simulink model "adaptive_lms1"  (Simulink 6.6)
settings: Solver=VariableStepDiscrete  StartTime=0.0  StopTime=15  RelTol=1e-3
StartFcn:
  | tic
StopFcn:
  | toc
libraries: dspbuff3 x2, simulink x2, dspwin32 x2, dspsigops x1, dspadpt3 x1
settings Model: Creator=lcrockett  LastModifiedBy=lcrockett
settings OptimizationCC: InlineParams=on  InlineInvariantSignals=on
settings DebuggingCC: SignalResolutionControl=TryResolveAllWithWarning  MultiTaskDSMMsg=warning  MultiTaskCondExecSysMsg=none  StrictBusMsg=None
settings HardwareCC: TargetHWDeviceType=32-bit Generic  ProdEqTarget=off
settings RTWCC: IncludeERTFirstTime=on

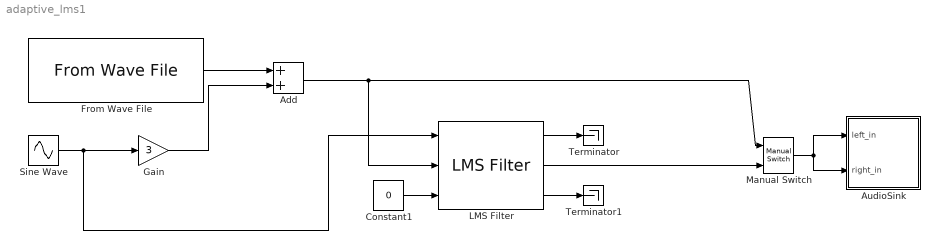
== system adaptive_lms1 ==
  Add : Sum  OutScaling=2^-10
  AudioSink : Subsystem
  Constant1 : Constant  Value=0
  From Wave File : dspwin32/From Wave File  FileName=Yabu_sample_48_mono  SamplesPerFrame=1  MinBufSize=1  dType=double  bLoop=off  timesToPlay=1  restartMode=immediately after last sample  firstSampleOutput=off  lastSampleOutput=off
  Gain : Gain  Gain=3
  LMS Filter : dspadpt3/LMS Filter  DialogController=dspDDGCreate  DialogControllerArgs=DataTag0  Algo=LMS  L=4  stepflag=Dialog  mu=0.001  leakage=1.0  ic=0  Adapt=off  resetflag=Non-zero sample  weights=on  secondCoeffMode=User-defined  secondCoeffWordLength=2  secondCoeffFracLength=15  accum2Mode=User-defined  accum2FracLength=20  prodOutput2Mode=User-defined  prodOutput2FracLength=20  prodOutput3Mode=User-defined  prodOutput3FracLength=20  prodOutput4Mode=User-defined  prodOutput4FracLength=20  quotientMode=User-defined  quotientFracLength=20  roundingMode=Floor  overflowMode=off  addnparflag=off
  Manual Switch : simulink/Signal Routing/Manual Switch  SystemSampleTime=-1  sw=0  action=0  varsize=off
  Sine Wave : Sin  Amplitude=0.5  Frequency=2*pi*1200  SampleTime=1/48000  VectorParams1D=off
  Terminator : Terminator
  Terminator1 : Terminator
  wires:
  From Wave File/1 -> Add/1
  Sine Wave/1 -> LMS Filter/1, Gain/1
  Manual Switch/1 -> AudioSink/1(left_in), AudioSink/2(right_in)
  Add/1 -> LMS Filter/2, Manual Switch/1
  LMS Filter/2 -> Manual Switch/2
  Gain/1 -> Add/2
  LMS Filter/1 -> Terminator/1
  LMS Filter/3 -> Terminator1/1
  Constant1/1 -> LMS Filter/3

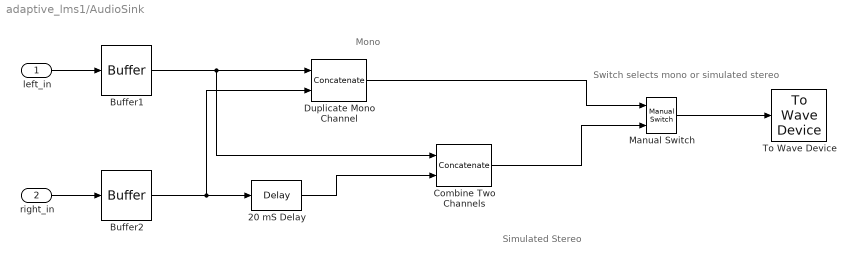
== system adaptive_lms1/AudioSink ==
  note: Mono
  note: Simulated
      | Stereo
  note: Switch selects mono
      | or simulated stereo
  left_in : Inport
  right_in : Inport  Port=2
  20 mS Delay : dspsigops/Delay  dly_unit=Samples  delay=20e-3 * 48000  ic_detail=on  dif_ic_for_ch=off  dif_ic_for_dly=off  ic=0  reset_popup=None
  Buffer1 : dspbuff3/Buffer  N=1  V=0  ic=0
  Buffer2 : dspbuff3/Buffer  N=1  V=0  ic=0
  Combine Two Channels : Concatenate  Mode=Multidimensional array  ConcatenateDimension=2
  Duplicate Mono Channel : Concatenate  Mode=Multidimensional array  ConcatenateDimension=2
  Manual Switch : simulink/Signal Routing/Manual Switch  SystemSampleTime=-1  sw=1  action=0  varsize=off
  To Wave Device : dspwin32/To Wave Device  bufDuration=0.1  determineBufSize=on  userIntBufSize=256  initDelay=0.1  useDefaultDevice=on  userDeviceID=SigmaTel Audio  enable24Bit=off
  wires:
  20 mS Delay/1 -> Combine Two Channels/2
  Duplicate Mono Channel/1 -> Manual Switch/1
  left_in/1 -> Buffer1/1
  Manual Switch/1 -> To Wave Device/1
  Combine Two Channels/1 -> Manual Switch/2
  right_in/1 -> Buffer2/1
  Buffer2/1 -> Duplicate Mono Channel/2, 20 mS Delay/1
  Buffer1/1 -> Duplicate Mono Channel/1, Combine Two Channels/1
